simulink model "controller"  (R2017a)
settings: Solver=FixedStepAuto  StartTime=0.0  StopTime=10.0  FixedStep=dt  RelTol=1e-3
values from neighbouring files (symbols this model uses):
  A = eye(6)    [PDController_Test.m]
  B = zeros(6,3)    [PDController_Test.m]
  D1 = 0*eye(3)    [PDController_Test.m]
  desired_state = [300, 300, 300, 0,0,0]'    [PDController_Test.m]
  K1 = 1*eye(3)    [PDController_Test.m]
  mass = 10    [PDController_Test.m]    (also in getG.m = 5; makeMatrixes.m = 1; testRobotDynamics.m)
settings Model: Creator=cibr-strokerehab  LastModifiedBy=cibr-strokerehab

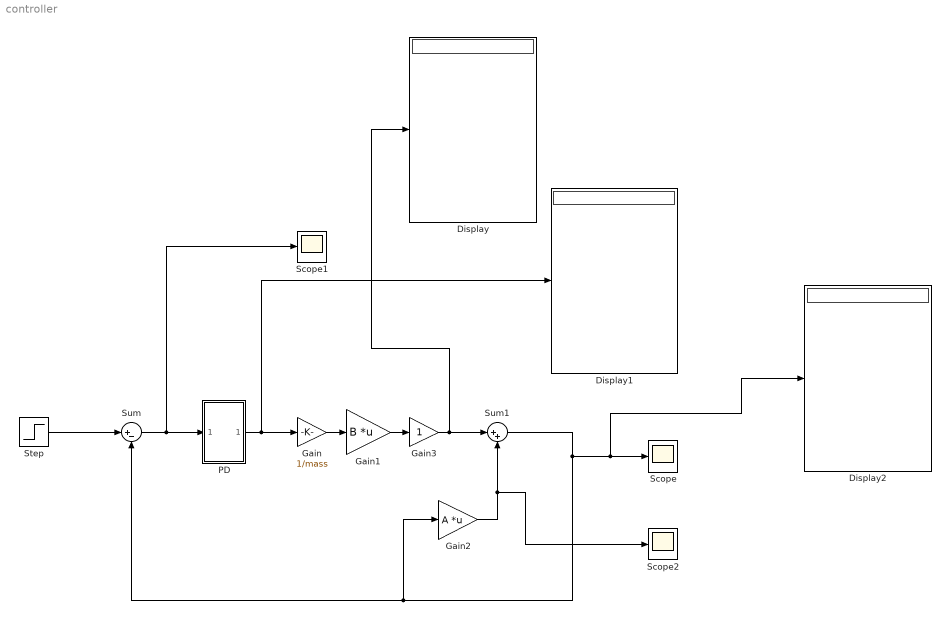
== system controller ==
  Display : Display
  Display1 : Display
  Display2 : Display
  Gain : Gain  Gain=1/mass
  Gain1 : Gain  Gain=B  Multiplication=Matrix(K*u)
  Gain2 : Gain  Gain=A  Multiplication=Matrix(K*u)
  Gain3 : Gain
  PD : Subsystem
  Scope : Scope
  Scope1 : Scope
  Scope2 : Scope
  Step : Step  Before=[0,0,0,0,0,0]'  After=desired_state  SampleTime=0
  Sum : Sum  Inputs=|+-
  Sum1 : Sum  Inputs=|++
  wires:
  PD/1(Out1) -> Gain/1, Display1/1
  Gain/1 -> Gain1/1
  Step/1 -> Sum/1
  Sum/1 -> Scope1/1, PD/1(In1)
  Sum1/1 -> Sum/2, Gain2/1, Display2/1, Scope/1
  Gain1/1 -> Gain3/1
  Gain2/1 -> Scope2/1, Sum1/2
  Gain3/1 -> Display/1, Sum1/1

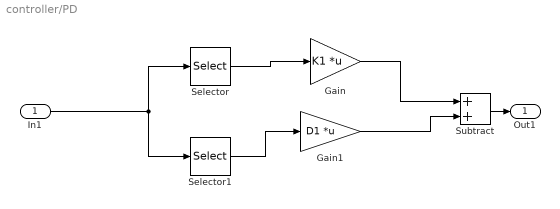
== system controller/PD ==
  In1 : Inport
  Gain : Gain  Gain=K1  Multiplication=Matrix(K*u)
  Gain1 : Gain  Gain=D1  Multiplication=Matrix(K*u)
  Selector : Selector  InputPortWidth=6  IndexOptions=Index vector (dialog)  Indices=[1 2 3]  OutputSizes=1
  Selector1 : Selector  InputPortWidth=6  IndexOptions=Index vector (dialog)  Indices=[4 5 6]  OutputSizes=1
  Subtract : Sum
  Out1 : Outport
  wires:
  Selector1/1 -> Gain1/1
  Gain1/1 -> Subtract/2
  In1/1 -> Selector1/1, Selector/1
  Subtract/1 -> Out1/1
  Selector/1 -> Gain/1
  Gain/1 -> Subtract/1
